simulink model "simulink4"  (R2025a)
settings: Solver=VariableStepAuto  StartTime=0.0  StopTime=10.0  RelTol=1e-3
settings Model: LastModifiedBy=ernes

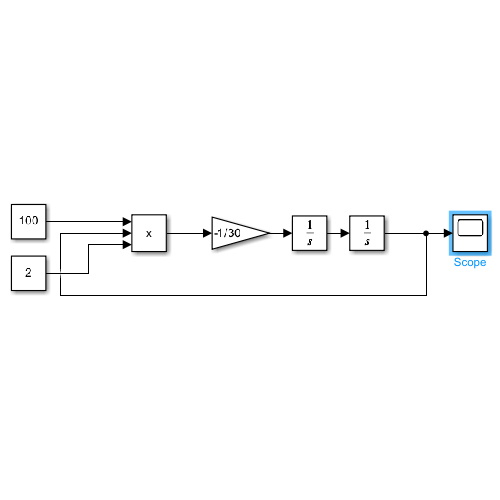
[thumbnail: Simulink's stored preview of the top-level diagram]
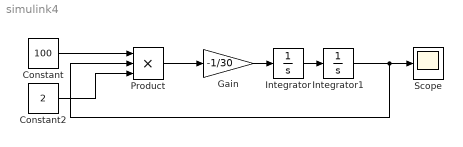
== system simulink4 ==
  Constant : Constant  Value=100
  Constant2 : Constant  Value=2
  Gain : Gain  Gain=-1/30
  Integrator : Integrator  InitialCondition=2
  Integrator1 : Integrator
  Product : Product  Inputs=3
  Scope : Scope
      settings: ActiveDisplayYMinimum=-0.96759548321980859  ActiveDisplayYMaximum=0.96805715405172021
  wires:
  Constant/1 -> Product/1
  Product/1 -> Gain/1
  Constant2/1 -> Product/3
  Integrator/1 -> Integrator1/1
  Integrator1/1 -> Product/2, Scope/1
  Gain/1 -> Integrator/1
